simulink model "lane_change"  (R2024a)
settings: Solver=VariableStepAuto  StartTime=0.0  StopTime=10.0  RelTol=1e-3
undefined symbols (not defined in the file): ids, ids_i, index_lane, route1_waypoint, route2_waypoint, route3_waypoint, route4_waypoint, route5_waypoint, waypoints, waypoints_i
libraries: CarMaker4SL x26
settings Model: Creator=User  LastModifiedBy=User

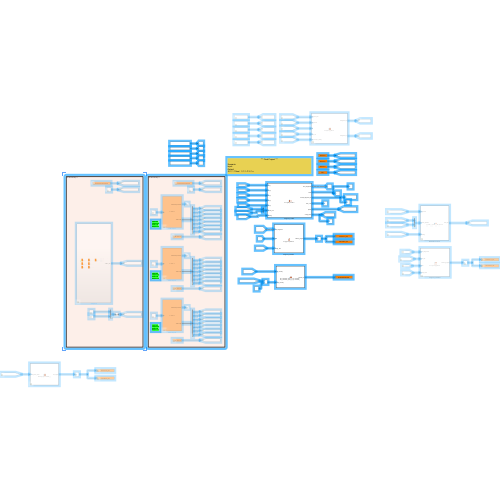
[thumbnail: Simulink's stored preview of the top-level diagram]
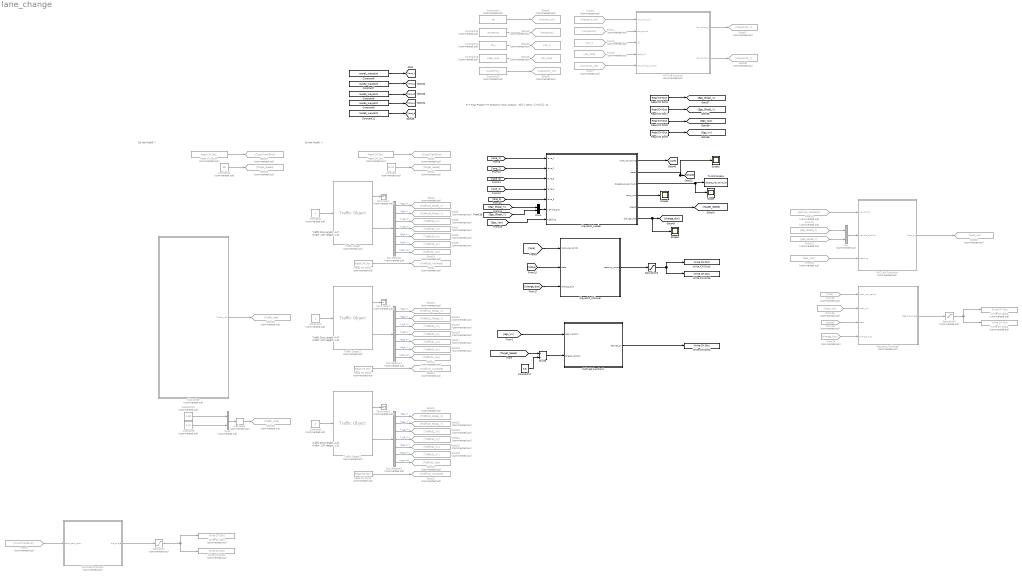
== system lane_change ==
  note: Traffic Size
      | Length: 4.47
      | Width: 1.97
      | Height: 1.12
  note: Do Not Modify !!
  note: *** Final Project ***
      |
      | Scenario:
      | Input:
      | Output:
      | 제어기 10ms / 다익스트라 1s
  note: Traffic Size
      | Length: 4.47
      | Width: 1.97
      | Height: 1.12
  note: Traffic Size
      | Length: 4.47
      | Width: 1.97
      | Height: 1.12
  note: Do Not Modify !!
  Bus Selector : BusSelector  Commented=on  OutputSignals=t_0 x,t_0 y,v_0 x,v_0 y,a_0 x,a_0 y,r_zyx z
  Bus Selector1 : BusSelector  Commented=on  OutputSignals=t_0 x,t_0 y,v_0 x,v_0 y,a_0 x,a_0 y,r_zyx z
  Bus Selector2 : BusSelector  Commented=on  OutputSignals=t_0 x,t_0 y,v_0 x,v_0 y,a_0 x,a_0 y,r_zyx z
  Constant : Constant  Commented=on  Value=22.22
  Constant1 : Constant  Commented=on  Value=0
  Constant10 : Constant  Commented=on  Value=2.48
  Constant11 : Constant  Value=route5_waypoint
  Constant12 : Constant  Commented=on  Value=ids
  Constant13 : Constant  Commented=on  Value=waypoints
  Constant14 : Constant  Commented=on  Value=ids_i
  Constant15 : Constant  Commented=on  Value=waypoints_i
  Constant16 : Constant  Commented=on  Value=index_lane
  Constant17 : Constant  Value=3.6
  Constant2 : Constant  Commented=on
  Constant3 : Constant  Commented=on  Value=2
  Constant4 : Constant  Commented=on  Value=80
  Constant5 : Constant  Commented=on  Value=11.5
  Constant6 : Constant  Value=route1_waypoint
  Constant7 : Constant  Value=route2_waypoint
  Constant8 : Constant  Value=route3_waypoint
  Constant9 : Constant  Value=route4_waypoint
  Divide : Product  Inputs=*/
  From1 : From  Commented=on  GotoTag=CrossTrackError
  From18 : From  Commented=on  GotoTag=optimal_cartesian
  From19 : From  Commented=on  GotoTag=state
  From21 : From  Commented=on  GotoTag=Ego_Global_X
  From22 : From  Commented=on  GotoTag=Ego_Gloabl_Y
  From23 : From  Commented=on  GotoTag=Ego_Yaw
  From24 : From  Commented=on  GotoTag=change_dist
  From25 : From  Commented=on  GotoTag=lane
  From26 : From  Commented=on  GotoTag=local_wp
  From3 : From  Commented=on  GotoTag=waypoint_idx
  From4 : From  Commented=on  GotoTag=waypoints
  From5 : From  Commented=on  GotoTag=idx_i
  From6 : From  Commented=on  GotoTag=idx_lane
  From7 : From  Commented=on  GotoTag=waypoints_idx
  Goto1 : Goto  Commented=on  GotoTag=CrossTrackError
  Goto10 : Goto  Commented=on  GotoTag=Traffic00_Yaw
  Goto11 : Goto  Commented=on  GotoTag=Traffic01_Yaw
  Goto12 : Goto  Commented=on  GotoTag=Traffic01_YawRate
  Goto13 : Goto  Commented=on  GotoTag=Traffic01_Global_X
  Goto14 : Goto  Commented=on  GotoTag=Traffic01_Global_Y
  Goto15 : Goto  Commented=on  GotoTag=Traffic01_Vx
  Goto16 : Goto  Commented=on  GotoTag=Traffic01_Vy
  Goto17 : Goto  Commented=on  GotoTag=Traffic01_Ax
  Goto18 : Goto  Commented=on  GotoTag=Traffic01_Ay
  Goto19 : Goto  Commented=on  GotoTag=Traffic02_Yaw
  Goto2 : Goto  Commented=on  GotoTag=Traffic00_YawRate
  Goto20 : Goto  Commented=on  GotoTag=Traffic02_YawRate
  Goto21 : Goto  Commented=on  GotoTag=Traffic02_Global_X
  Goto22 : Goto  Commented=on  GotoTag=Traffic02_Global_Y
  Goto23 : Goto  Commented=on  GotoTag=Traffic02_Vx
  Goto24 : Goto  Commented=on  GotoTag=Traffic02_Vy
  Goto25 : Goto  Commented=on  GotoTag=Traffic02_Ax
  Goto26 : Goto  Commented=on  GotoTag=Traffic02_Ay
  Goto27 : Goto  Commented=on  GotoTag=CrossTrackError
  Goto28 : Goto  Commented=on  GotoTag=Traffic_size
  Goto29 : Goto  Commented=on  GotoTag=Target_Speed
  Goto3 : Goto  Commented=on  GotoTag=Traffic00_Global_X
  Goto30 : Goto  Commented=on  GotoTag=Traffic_Info
  Goto4 : Goto  Commented=on  GotoTag=Target_Speed
  Goto42 : Goto  Commented=on  GotoTag=waypint_idx
  Goto43 : Goto  Commented=on  GotoTag=waypoints
  Goto44 : Goto  Commented=on  GotoTag=idx_i
  Goto45 : Goto  Commented=on  GotoTag=idx_lane
  Goto46 : Goto  Commented=on  GotoTag=waypoints_idx
  Goto47 : Goto  Commented=on  GotoTag=Waypoints_X
  Goto48 : Goto  Commented=on  GotoTag=Waypoints_Y
  Goto5 : Goto  Commented=on  GotoTag=Traffic00_Global_Y
  Goto50 : Goto  Commented=on  GotoTag=local_wp
  Goto6 : Goto  Commented=on  GotoTag=Traffic00_Vx
  Goto7 : Goto  Commented=on  GotoTag=Traffic00_Vy
  Goto8 : Goto  Commented=on  GotoTag=Traffic00_Ax
  Goto9 : Goto  Commented=on  GotoTag=Traffic00_Ay
  MATLAB Function : MATLAB Function  Commented=on  TreatAsAtomicUnit=on
  MATLAB Function1 : MATLAB Function  TreatAsAtomicUnit=on
  MATLAB Function2 : MATLAB Function  Commented=on  TreatAsAtomicUnit=on
  "MATLAB Function4 " : MATLAB Function  Commented=on  TreatAsAtomicUnit=on
  Mux : Mux  Commented=on  Inputs=2
  Mux1 : Mux  Inputs=2
  Mux3 : Mux  Commented=on  Inputs=2
  Read CM Dict : CarMaker4SL/Read CM Dict  Commented=on  xname=Car.Road.Path.DevDist  xsync=off  xstime=Inherited
  Read CM Dict1 : CarMaker4SL/Read CM Dict  Commented=on  xname=Traffic.T22.rzv  xsync=off  xstime=Inherited
  Read CM Dict2 : CarMaker4SL/Read CM Dict  Commented=on  xname=Traffic.T23.rzv  xsync=off  xstime=Inherited
  Read CM Dict3 : CarMaker4SL/Read CM Dict  Commented=on  xname=Traffic.T24.rzv  xsync=off  xstime=Inherited
  Read CM Dict4 : CarMaker4SL/Read CM Dict  Commented=on  xname=Car.Road.Path.DevDist  xsync=off  xstime=Inherited
  Read CM Dict6 : CarMaker4SL/Read CM Dict  xname=Car.Fr1.tx  xsync=off  xstime=Inherited
  Read CM Dict7 : CarMaker4SL/Read CM Dict  xname=Car.Fr1.ty  xsync=off  xstime=Inherited
  Read CM Dict8 : CarMaker4SL/Read CM Dict  xname=Car.Fr1.rz  xsync=off  xstime=Inherited
  Read CM Dict9 : CarMaker4SL/Read CM Dict  xname=Car.v  xsync=off  xstime=Inherited
  Reshape1 : Reshape  Commented=on  OutputDimensionality=Row vector (2-D)  OutputDimensions=[2,2]
  Saturation : Saturate  Commented=on  UpperLimit=2  LowerLimit=-2
  Saturation1 : Saturate  Commented=on  UpperLimit=2  LowerLimit=-2
  Saturation2 : Saturate  UpperLimit=2  LowerLimit=-2
  Scope{,1..3} (4 alike) : Scope
  Subsystem : Subsystem  Commented=on
  Terminator : Terminator  Commented=on
  Terminator1 : Terminator  Commented=on
  Terminator2 : Terminator  Commented=on
  To Workspace : ToWorkspace  VariableName=closest_waypoint_idx  SaveFormat=Structure With Time  SampleTime=-1
  Traffic Object : CarMaker4SL/Traffic Object  Commented=on  xname=T00  ximode=Traffic Id  xstime=Inherited
      settings: SourceProductName=CarMaker4SL
  Traffic Object1 : CarMaker4SL/Traffic Object  Commented=on  xname=T01  ximode=Traffic Id  xstime=Inherited
      settings: SourceProductName=CarMaker4SL
  Traffic Object2 : CarMaker4SL/Traffic Object  Commented=on  xname=T02  ximode=Traffic Id  xstime=Inherited
      settings: SourceProductName=CarMaker4SL
  Waypoint_Follower : MATLAB Function  TreatAsAtomicUnit=on
  Waypoint_Follower1 : MATLAB Function  Commented=on  TreatAsAtomicUnit=on
  Waypoint_Loader : MATLAB Function  TreatAsAtomicUnit=on
  Write CM Dict : CarMaker4SL/Write CM Dict  Commented=on  xname=Car.CFL.rz_ext  xsync=off
  Write CM Dict1 : CarMaker4SL/Write CM Dict  Commented=on  xname=Car.CFR.rz_ext  xsync=off
  Write CM Dict2 : CarMaker4SL/Write CM Dict  xname=AccelCtrl.DesiredAx  xsync=off
  Write CM Dict3 : CarMaker4SL/Write CM Dict  Commented=on  xname=Car.CFL.rz_ext  xsync=off
  Write CM Dict4 : CarMaker4SL/Write CM Dict  Commented=on  xname=Car.CFR.rz_ext  xsync=off
  Write CM Dict5 : CarMaker4SL/Write CM Dict  xname=Car.CFL.rz_ext  xsync=off
  Write CM Dict6 : CarMaker4SL/Write CM Dict  xname=Car.CFR.rz_ext  xsync=off
  wires:
  "MATLAB Function4 "/1(local_wp) -> Goto50/1
  From21/1 -> Mux/1
  Mux/1 -> "MATLAB Function4 "/2(vehicle_position)
  From18/1 -> "MATLAB Function4 "/1(waypoints)
  From22/1 -> Mux/2
  From25/1 -> Waypoint_Follower1/1(local_waypoints)
  From23/1 -> "MATLAB Function4 "/3(heading)
  Saturation1/1 -> Write CM Dict3/1, Write CM Dict4/1
  From19/1 -> Waypoint_Follower1/3(state)
  Waypoint_Follower1/1(steering_angle) -> Saturation1/1
  From24/1 -> Waypoint_Follower1/4(change_dist)
  From26/1 -> Waypoint_Follower1/2(local_wp)
  Waypoint_Loader/6(change_dist) -> Scope3/1, [change_dist]
  [change_dist] -> Waypoint_Follower/3(change_dist)
  Waypoint_Loader/3(closest_waypoint_idx) -> Scope/1, To Workspace/1
  Constant17/1 -> Divide/2
  Divide/1 -> MATLAB Function1/2(target_velocity)
  [Target_Speed] -> Divide/1
  Traffic Object1/1 -> Terminator1/1
  Waypoint_Loader/4(lane_num) -> Scope1/1
  Constant15/1 -> Goto46/1
  From5/1 -> MATLAB Function/3(idx)
  Bus Selector2/7 -> Goto19/1  "<r_zyx z>"
  [state] -> Waypoint_Follower/2(state)
  Waypoint_Loader/5(speed) -> [Target_Speed]
  Waypoint_Loader/2(state) -> Scope2/1, [state]
  Waypoint_Follower/1(steering_angle) -> Saturation2/1
  From3/1 -> MATLAB Function/1(waypoint_idx)
  Mux3/1 -> Reshape1/1
  [lane] -> Waypoint_Follower/1(local_waypoints)
  [lane_2] -> Waypoint_Loader/2(lane_2)
  Read CM Dict/1 -> Goto1/1
  Constant9/1 -> [lane_4]
  Bus Selector1/1 -> Goto13/1  "<t_0 x>"
  Traffic Object1/2 -> Bus Selector1/1
  Bus Selector/6 -> Goto9/1  "<a_0 y>"
  [Ego_Gloabl_Y] -> Mux1/2
  Constant7/1 -> [lane_2]
  [lane_3] -> Waypoint_Loader/3(lane_3)
  [lane_5] -> Waypoint_Loader/5(lane_5)
  [lane_4] -> Waypoint_Loader/4(lane_4)
  Bus Selector/4 -> Goto7/1  "<v_0 y>"
  Mux1/1 -> Waypoint_Loader/6(vehicle_pos)
  Bus Selector1/2 -> Goto14/1  "<t_0 y>"
  [Ego_Vx] -> MATLAB Function1/1(ego_velocity)
  Constant3/1 -> Traffic Object2/1
  Constant8/1 -> [lane_3]
  [lane_1] -> Waypoint_Loader/1(lane_1)
  Traffic Object/1 -> Terminator/1
  Bus Selector1/3 -> Goto15/1  "<v_0 x>"
  Bus Selector2/3 -> Goto23/1  "<v_0 x>"
  Saturation2/1 -> Write CM Dict5/1, Write CM Dict6/1
  MATLAB Function1/1(desired_ax) -> Write CM Dict2/1
  Read CM Dict8/1 -> [Ego_Yaw]
  Read CM Dict9/1 -> [Ego_Vx]
  Constant14/1 -> Goto44/1
  Constant16/1 -> Goto45/1
  MATLAB Function/2(Waypoints_Y) -> Goto48/1
  Constant4/1 -> Goto29/1
  Bus Selector/7 -> Goto10/1  "<r_zyx z>"
  Constant6/1 -> [lane_1]
  Saturation/1 -> Write CM Dict/1, Write CM Dict1/1
  MATLAB Function/1(Waypoints_X) -> Goto47/1
  From6/1 -> MATLAB Function/4(lane_idx)
  Bus Selector2/2 -> Goto22/1  "<t_0 y>"
  From4/1 -> MATLAB Function/2(waypoints)
  Read CM Dict6/1 -> [Ego_Global_X]
  Read CM Dict7/1 -> [Ego_Gloabl_Y]
  Bus Selector2/4 -> Goto24/1  "<v_0 y>"
  Bus Selector1/7 -> Goto11/1  "<r_zyx z>"
  Reshape1/1 -> Goto28/1
  From7/1 -> MATLAB Function/5(waypoints_id_array)
  Subsystem/1(Traffic_Info) -> Goto30/1
  Waypoint_Loader/1(local_waypoints) -> [lane]
  Bus Selector1/4 -> Goto16/1  "<v_0 y>"
  Read CM Dict4/1 -> Goto27/1
  Bus Selector2/5 -> Goto25/1  "<a_0 x>"
  Bus Selector1/6 -> Goto18/1  "<a_0 y>"
  Constant13/1 -> Goto43/1
  Traffic Object2/1 -> Terminator2/1
  Traffic Object2/2 -> Bus Selector2/1
  Constant10/1 -> Mux3/1
  Constant11/1 -> [lane_5]
  Constant1/1 -> Traffic Object/1
  [Ego_Yaw] -> Waypoint_Loader/7(heading)
  Constant2/1 -> Traffic Object1/1
  Constant5/1 -> Mux3/2
  Bus Selector2/6 -> Goto26/1  "<a_0 y>"
  Bus Selector2/1 -> Goto21/1  "<t_0 x>"
  Bus Selector/1 -> Goto3/1  "<t_0 x>"
  Bus Selector/3 -> Goto6/1  "<v_0 x>"
  Constant/1 -> Goto4/1
  Read CM Dict3/1 -> Goto20/1
  Read CM Dict1/1 -> Goto2/1
  Bus Selector1/5 -> Goto17/1  "<a_0 x>"
  Read CM Dict2/1 -> Goto12/1
  Bus Selector/5 -> Goto8/1  "<a_0 x>"
  Constant12/1 -> Goto42/1
  MATLAB Function2/1(tire_angle) -> Saturation/1
  Traffic Object/2 -> Bus Selector/1
  [Ego_Global_X] -> Mux1/1
  From1/1 -> MATLAB Function2/1(cross_track_error)
  Bus Selector/2 -> Goto5/1  "<t_0 y>"

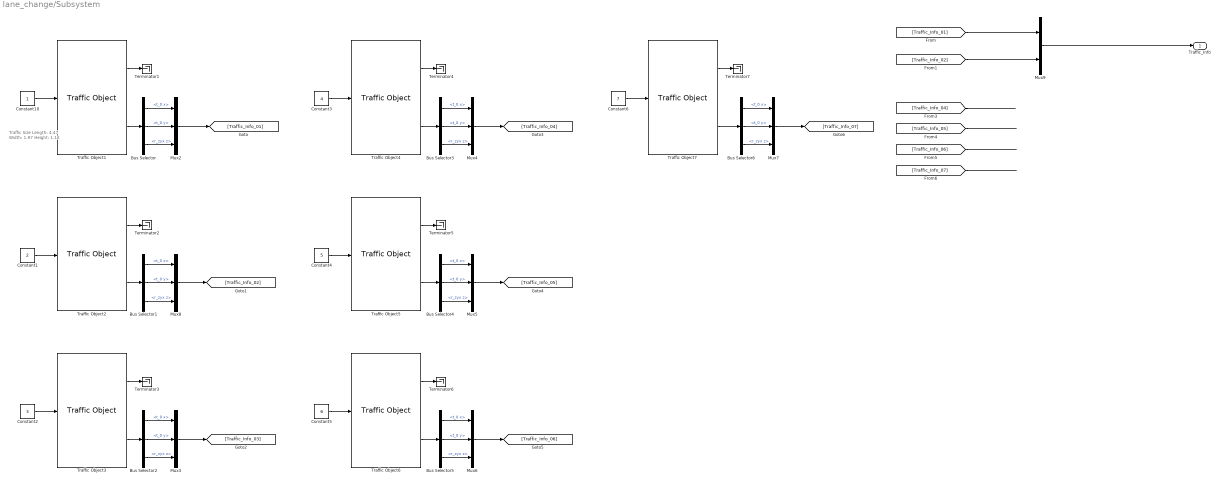
== system lane_change/Subsystem ==
  note: Traffic Size
      | Length: 4.47
      | Width: 1.97
      | Height: 1.12
  Bus Selector{,1..6} (7 alike) : BusSelector  OutputSignals=t_0 x,t_0 y,r_zyx z
  Constant1 : Constant  Value=2
  Constant10 : Constant
  Constant2 : Constant  Value=3
  Constant3 : Constant  Value=4
  Constant4 : Constant  Value=5
  Constant5 : Constant  Value=6
  Constant6 : Constant  Value=7
  Mux{2..8} (7 alike) : Mux  Inputs=3
  Mux9 : Mux  Inputs=2
  Terminator{1..7} (7 alike) : Terminator
  Traffic Object1 : CarMaker4SL/Traffic Object  xname=T01  ximode=Traffic Id  xstime=Inherited
      settings: SourceProductName=CarMaker4SL
  Traffic Object2 : CarMaker4SL/Traffic Object  xname=T02  ximode=Traffic Id  xstime=Inherited
      settings: SourceProductName=CarMaker4SL
  Traffic Object3 : CarMaker4SL/Traffic Object  xname=T03  ximode=Traffic Id  xstime=Inherited
      settings: SourceProductName=CarMaker4SL
  Traffic Object4 : CarMaker4SL/Traffic Object  xname=T04  ximode=Traffic Id  xstime=Inherited
      settings: SourceProductName=CarMaker4SL
  Traffic Object5 : CarMaker4SL/Traffic Object  xname=T05  ximode=Traffic Id  xstime=Inherited
      settings: SourceProductName=CarMaker4SL
  Traffic Object6 : CarMaker4SL/Traffic Object  xname=T06  ximode=Traffic Id  xstime=Inherited
      settings: SourceProductName=CarMaker4SL
  Traffic Object7 : CarMaker4SL/Traffic Object  xname=T07  ximode=Traffic Id  xstime=Inherited
      settings: SourceProductName=CarMaker4SL
  Traffic_Info : Outport
  wires:
  Constant10/1 -> Traffic Object1/1
  Traffic Object1/1 -> Terminator1/1
  Traffic Object2/1 -> Terminator2/1
  Constant1/1 -> Traffic Object2/1
  Constant2/1 -> Traffic Object3/1
  Traffic Object3/1 -> Terminator3/1
  Traffic Object4/1 -> Terminator4/1
  Constant3/1 -> Traffic Object4/1
  Constant4/1 -> Traffic Object5/1
  Traffic Object5/1 -> Terminator5/1
  Traffic Object6/1 -> Terminator6/1
  Constant5/1 -> Traffic Object6/1
  Constant6/1 -> Traffic Object7/1
  Traffic Object7/1 -> Terminator7/1
  [Traffic_Info_04] -> ?
  [Traffic_Info_05] -> ?
  [Traffic_Info_06] -> ?
  [Traffic_Info_07] -> ?
  Traffic Object1/2 -> Bus Selector/1
  Bus Selector/1 -> Mux2/1  "<t_0 x>"
  Bus Selector/2 -> Mux2/2  "<t_0 y>"
  Bus Selector/3 -> Mux2/3  "<r_zyx z>"
  Bus Selector1/2 -> Mux8/2  "<t_0 y>"
  Mux8/1 -> [Traffic_Info_02]
  Bus Selector1/1 -> Mux8/1  "<t_0 x>"
  Bus Selector1/3 -> Mux8/3  "<r_zyx z>"
  Traffic Object2/2 -> Bus Selector1/1
  Bus Selector2/2 -> Mux3/2  "<t_0 y>"
  Mux3/1 -> [Traffic_Info_03]
  Bus Selector2/1 -> Mux3/1  "<t_0 x>"
  Bus Selector2/3 -> Mux3/3  "<r_zyx z>"
  Traffic Object3/2 -> Bus Selector2/1
  Bus Selector3/2 -> Mux4/2  "<t_0 y>"
  Mux4/1 -> [Traffic_Info_04]
  Bus Selector3/1 -> Mux4/1  "<t_0 x>"
  Bus Selector3/3 -> Mux4/3  "<r_zyx z>"
  Traffic Object4/2 -> Bus Selector3/1
  Bus Selector4/2 -> Mux5/2  "<t_0 y>"
  Mux5/1 -> [Traffic_Info_05]
  Bus Selector4/1 -> Mux5/1  "<t_0 x>"
  Bus Selector4/3 -> Mux5/3  "<r_zyx z>"
  Traffic Object5/2 -> Bus Selector4/1
  Bus Selector5/2 -> Mux6/2  "<t_0 y>"
  Mux6/1 -> [Traffic_Info_06]
  Bus Selector5/1 -> Mux6/1  "<t_0 x>"
  Bus Selector5/3 -> Mux6/3  "<r_zyx z>"
  Traffic Object6/2 -> Bus Selector5/1
  Bus Selector6/2 -> Mux7/2  "<t_0 y>"
  Mux7/1 -> [Traffic_Info_07]
  Bus Selector6/1 -> Mux7/1  "<t_0 x>"
  Bus Selector6/3 -> Mux7/3  "<r_zyx z>"
  Traffic Object7/2 -> Bus Selector6/1
  Mux2/1 -> [Traffic_Info_01]
  [Traffic_Info_01] -> Mux9/1
  [Traffic_Info_02] -> Mux9/2
  Mux9/1 -> Traffic_Info/1

== matlab function lane_change/MATLAB Function4  ==
  settings: sampleTime=0.1
  data: waypoints input; local_wp output; vehicle_position input; heading input
function local_wp = global_to_local_waypoints(waypoints, vehicle_position, heading)

    waypoints_x = waypoints(:,1);
    waypoints_y = waypoints(:,2);
    num_points = length(waypoints_x);

    local_wp = zeros(num_points, 2);
    x_ego = vehicle_position(1);
    y_ego = vehicle_position(2);
    
    for i = 1:num_points
        dx = waypoints_x(i) - x_ego;
        dy = waypoints_y(i) - y_ego;

        local_x = dx * cos(-heading) - dy * sin(-heading);
        local_y = dx * sin(-heading) + dy * cos(-heading);

        local_wp(i, :) = [local_x, local_y];
    end    
end

== matlab function lane_change/Waypoint_Loader ==
  data: lane_1 input; local_waypoints output; lane_2 input; lane_3 input; lane_4 input; lane_5 input; state output; vehicle_pos input; heading input; closest_waypoint_idx output; lane_num output; speed output; change_dist output
function [local_waypoints, state, closest_waypoint_idx, lane_num, speed, change_dist] = waypoint_loader(lane_1, lane_2, lane_3, lane_4, lane_5, vehicle_pos, heading)
    
    lane_5 = [lane_5; 2.38, -36.18; 3.17, -36.47; 4, -36.6; 4.5, -36.6; 5.0, -36.6; 5.5, -36.6];

    persistent lap_count;
    if isempty(lap_count)
        lap_count = 1;
    end
    persistent entry_5;
    if isempty(entry_5)
        entry_5 = 1;
    end

    lane = lane_2; 
    state = 0;
    lane_num = 0;
    speed = 0;
    change_dist = 0;

    distances = sqrt((lane(:,1) - vehicle_pos(1)).^2 + (lane(:,2) - vehicle_pos(2)).^2);
    [~, closest_waypoint_idx] = min(distances);

    if lap_count == 1
        if closest_waypoint_idx < 18
            lane = lane_2;
            lane_num = 2;
            speed = 50;
        elseif closest_waypoint_idx < 55
            lane = lane_1;
            lane_num = 1;
            speed = 50;
        elseif closest_waypoint_idx < 87
            lane = lane_2;
            lane_num = 2;
            speed = 50;
        elseif closest_waypoint_idx < 125
            lane = lane_1;
            lane_num = 1;
            speed = 50;
        elseif closest_waypoint_idx < 180
            lane = lane_2;
            lane_num = 2;
            state = 0;
            speed = 50;
        elseif closest_waypoint_idx < 190
            lane = lane_1;
            lane_num = 1;
            state = 1;
            speed = 50;
        elseif closest_waypoint_idx < 200
            lane = lane_2;
            lane_num = 2;
            state = 2;
            speed = 50;
        elseif closest_waypoint_idx < 224
            lane = lane_3;
            lane_num = 3;
            state = 3;
            speed = 50;
            lap_count = lap_count + 1;
        else
            lane = lane_2;
            lane_num = 2;
            speed = 50;
        end


    else
        lane = lane_3;
        if closest_waypoint_idx < 9
            lane = lane_3;
            lane_num = 50;
            state = 5;
            speed = 50;
        elseif closest_waypoint_idx < 22
            lane = lane_4;
            lane_num = 80;
            speed = 30;
            entry_5 = entry_5 + 1;
            state = 6;
        elseif entry_5 > 1
            lane = lane_5;
            lane_num = 200;
            state = 7;
            speed = 10;
        else 
            lane = lane_3;
            lane_num = 100; 
            state = 4;
            speed = 50;
        end
    end

    % closest_waypoint 
    distances = sqrt((lane(:,1) - vehicle_pos(1)).^2 + (lane(:,2) - vehicle_pos(2)).^2);
    [~, closest_waypoint_idx] = min(distances);
    start_idx = closest_waypoint_idx;
    
    % lane_change diff dist
    dx_c = lane(closest_waypoint_idx, 1) - vehicle_pos(1);
    dy_c = lane(closest_waypoint_idx, 2) - vehicle_pos(2);
    change_dist = sqrt(dx_c^2 + dy_c^2);

    % 10 waypoint select
    end_idx = min(start_idx + 9, size(lane, 1));
    selected_waypoints = lane(start_idx:end_idx, :);

    % local transform
    local_waypoints = zeros(size(selected_waypoints));
    for i = 1:size(selected_waypoints, 1)
        dx = selected_waypoints(i, 1) - vehicle_pos(1);
        dy = selected_waypoints(i, 2) - vehicle_pos(2);

        local_x = dx * cos(-heading) - dy * sin(-heading);
        local_y = dx * sin(-heading) + dy * cos(-heading);

        local_waypoints(i, :) = [local_x, local_y];
    end
end

% function [local_waypoints, state, closest_waypoint_idx, lane_num] = waypoint_loader(lane_1, lane_2, lane_3, lane_4, lane_5, vehicle_pos, heading)
% 
%     persistent lap_count current_lane_num;
%     if isempty(lap_count)
%         lap_count = 1;
%     end
% 
%     if isempty(current_lane_num)
%         current_lane_num = 2;
%     end
% 
%     lane_list = {lane_1, lane_2, lane_3, lane_4, lane_5};
% 
%     current_lane = lane_list{current_lane_num};
%     distances = sqrt((current_lane(:,1) - vehicle_pos(1)).^2 + (current_lane(:,2) - vehicle_pos(2)).^2);
%     [~, closest_waypoint_idx] = min(distances);
% 
%     if lap_count == 1
%         if  closest_waypoint_idx > 200
%             current_lane_num = 1; 
%         elseif closest_waypoint_idx > 210
%             current_lane_num = 2; 
%         elseif  closest_waypoint_idx > 223
%             current_lane_num = 3;
%             lap_count = lap_count + 1;
%         else 
%             current_lane_num = 2;
%         end
%     else
%         % --- Lap 2 이상 로직 ---
%         if current_lane_num == 3 && closest_waypoint_idx > 10
%             current_lane_num = 4;
%         elseif current_lane_num == 4 && closest_waypoint_idx > 15
%             current_lane_num = 5;
%         end
%     end
% 
%     % 최종 lane 정보
%     lane = lane_list{current_lane_num};
%     lane_num = current_lane_num;
% 
%     % 최신 lane에 대해 closest waypoint 재계산
%     distances = sqrt((lane(:,1) - vehicle_pos(1)).^2 + (lane(:,2) - vehicle_pos(2)).^2);
%     [~, closest_waypoint_idx] = min(distances);
% 
% 
%     start_idx = closest_waypoint_idx;
%     end_idx = min(start_idx + 9, size(lane, 1));
%     selected_waypoints = lane(start_idx:end_idx, :);
% 
%     local_waypoints = zeros(size(selected_waypoints));
%     for i = 1:size(selected_waypoints, 1)
%         dx = selected_waypoints(i, 1) - vehicle_pos(1);
%         dy = selected_waypoints(i, 2) - vehicle_pos(2);
% 
%         local_x = dx * cos(-heading) - dy * sin(-heading);
%         local_y = dx * sin(-heading) + dy * cos(-heading);
% 
%         local_waypoints(i, :) = [local_x, local_y];
%     end
% 
%     state = 0; % 필요에 따라 갱신
% 
% end

== matlab function lane_change/MATLAB Function ==
  data: Waypoints_X output; waypoint_idx input; waypoints input; idx input; lane_idx input; waypoints_id_array input; Waypoints_Y output
function [Waypoints_X, Waypoints_Y]  = waypoint_loader(waypoint_idx, waypoints, idx, lane_idx, waypoints_id_array)

% 초기화
Waypoints_X = zeros(1, 50);  % 1번 lane은 최대 50개라고 가정
Waypoints_Y = zeros(1, 50);

% 1번 lane만 출력
target_lane = 1;

for i = 1:length(idx)
    if lane_idx(i) == target_lane
        % 현재 row가 target_lane에 해당함
        waypoint_ids = waypoints_id_array(i, :);  % 1x50 인덱스 추출
        for j = 1:50
            wp_id = waypoint_ids(j);
            if wp_id > 0 && wp_id <= size(waypoints, 1)
                Waypoints_X(j) = waypoints(wp_id, 1);
                Waypoints_Y(j) = waypoints(wp_id, 2);
            end
        end
        break;  % 1번 lane 하나만 처리하면 되므로 종료
    end
end

== matlab function lane_change/Waypoint_Follower1 ==
  settings: sampleTime=0.1
  data: local_waypoints input; local_wp input; steering_angle output; state input; change_dist input
% local tracking
function steering_angle = waypoint_follower(local_waypoints, local_wp, state, change_dist)

    WHEEL_BASE = 2.9;
    lookahead_dist = 4.5;

    if((state == 1 || state == 2 || state == 3 || state == 4))
        lookahead_dist = 10;
    end

    if(state == 7)
        lookahead_dist = 2.5;
    end

    target_idx = -1;
    final_ld = 0;

    for i = 1:size(local_waypoints, 1)
        dist = norm(local_waypoints(i, :));
        if dist > lookahead_dist && local_waypoints(i, 1) > 0
            target_idx = i;
            final_ld = dist;
            break;
        end
    end

    if target_idx == -1
        steering_angle = 0;
        return;
    end

    target_point = local_waypoints(target_idx, :);
    alpha = atan2(target_point(2), target_point(1));
    alpha = wrapToPi(alpha);

    final_ld = min(max(final_ld, 2.0), 20.0); 

    steering_angle = atan2(2 * WHEEL_BASE * sin(alpha), final_ld);
end

== matlab function lane_change/MATLAB Function1 ==
  settings: sampleTime=0.1
  data: ego_velocity input; desired_ax output; target_velocity input
function desired_ax = longitudinal_speed_pid_controller_(ego_velocity, target_velocity)
    persistent Kp Kd prev_error dt

    % 초기화 (한 번만 실행)
    if isempty(prev_error)
        Kp = 1.0;     % 비례 이득
        Kd = 0.0;     % 미분 이득
        dt = 0.001;    % 제어 주기 (초)
        prev_error = 0;
    end

    % 오차 계산
    error = target_velocity - ego_velocity;
    d_error = (error - prev_error) / dt;

    % PD 제어 계산
    desired_ax = Kp * error + Kd * d_error;

    % 상태 업데이트
    prev_error = error;
end

== matlab function lane_change/MATLAB Function2 ==
  settings: sampleTime=0.1
  data: cross_track_error input; tire_angle output
function tire_angle = lateral_pid_controller_(cross_track_error)
    persistent prev_error Kp Kd dt

    % 초기화 (첫 호출 시 한 번만 실행)
    if isempty(prev_error)
        prev_error = 0;
        dt = 0.001;   % 제어 주기 (초)
        Kp = 0.1;     % 비례 이득 (튜닝 가능)
        Kd = 0.004;    % 미분 이득 (튜닝 가능)
    end

    % 오차 변화율 계산
    d_error = (cross_track_error - prev_error) / dt;

    % PD 제어 계산
    tire_angle = -Kp * cross_track_error - Kd * d_error;


    % 상태 업데이트
    prev_error = cross_track_error;
end

== matlab function lane_change/Waypoint_Follower ==
  settings: sampleTime=0.1
  data: local_waypoints input; steering_angle output; state input; change_dist input
% local tracking
function steering_angle = waypoint_follower(local_waypoints, state, change_dist)

    WHEEL_BASE = 2.9;
    lookahead_dist = 4.5;
    
    % sigmoid lookahead_dist change
    if(change_dist > 1.8) 
        lookahead_dist = (10 / (1 + exp(-0.4 * change_dist))) + 5;
    end

    % final state -> parking area entry
    if(state == 7)
        lookahead_dist = 2.5;
    end

    target_idx = -1;
    final_ld = 0;

    for i = 1:size(local_waypoints, 1)
        dist = norm(local_waypoints(i, :));
        if dist > lookahead_dist && local_waypoints(i, 1) > 0
            target_idx = i;
            final_ld = dist;
            break;
        end
    end

    if target_idx == -1
        steering_angle = 0;
        return;
    end

    target_point = local_waypoints(target_idx, :);
    alpha = atan2(target_point(2), target_point(1));
    alpha = wrapToPi(alpha);

    final_ld = min(max(final_ld, 2.0), 20.0); 

    steering_angle = atan2(2 * WHEEL_BASE * sin(alpha), final_ld);
end


% % global tracking
% function [steering_angle, start_idx] = pure_pursuit(waypoints, vehicle_position, head)
% 
%     persistent last_target_idx;
%     if isempty(last_target_idx)
%         last_target_idx = 1; % 초기값 설정
%     end
% 
%     WHEEL_BASE = 2.7;
% 
%     waypoints_x = waypoints(:,1);
%     waypoints_y = waypoints(:,2);
%     % num_points = length(waypoints_x);
%     num_points = 300;
% 
%     local_waypoints = zeros(num_points, 2);
%     x_ego = vehicle_position(1);
%     y_ego = vehicle_position(2);
% 
%     for i = 1:num_points
%         dx = waypoints_x(i) - x_ego;
%         dy = waypoints_y(i) - y_ego;
% 
%         local_x = dx * cos(-head) - dy * sin(-head);
%         local_y = dx * sin(-head) + dy * cos(-head);
% 
%         local_waypoints(i, :) = [local_x, local_y];
%     end    
% 
%     lookahead_dist = 5.0;
% 
%     distances_to_waypoints = sqrt((waypoints_x - x_ego).^2 + (waypoints_y - y_ego).^2);
%     [~, closest_idx] = min(distances_to_waypoints);
% 
%     start_idx = max(last_target_idx, closest_idx);
% 
%     target_idx = -1;
%     final_ld = 0;
%     for i = start_idx:num_points
%         dist = norm(local_waypoints(i, :));
%         if dist > lookahead_dist && local_waypoints(i, 1) > 0
%             target_idx = i;
%             final_ld = dist;
%             break;
%         end
%     end
% 
%     if target_idx == -1
%         for i = 1:start_idx-1
%             dist = norm(local_waypoints(i, :));
%             if dist > lookahead_dist && local_waypoints(i, 1) > 0
%                 target_idx = i;
%                 final_ld = dist;
%                 break;
%             end
%         end
%     end
% 
%     if target_idx == -1
%         steering_angle = 0;
%         return;
%     end
% 
%     target_point = local_waypoints(target_idx, :);
%     alpha = atan2(target_point(2), target_point(1));
%     alpha = wrapToPi(alpha);
% 
%     final_ld = min(max(final_ld, 2.0), 20.0);
% 
%     steering_angle = atan2(2 * WHEEL_BASE * sin(alpha), final_ld);
% 
%     last_target_idx = target_idx;
% end
